simulink model "carPlant_GeHumanFollower"  (R2018b)
settings: Solver=VariableStepAuto  StartTime=0.0  StopTime=20  RelTol=1e-3
libraries: autolibshared x2, vehdynlibsteering x2
settings Model: Creator=ckreienk  LastModifiedBy=ckreienk

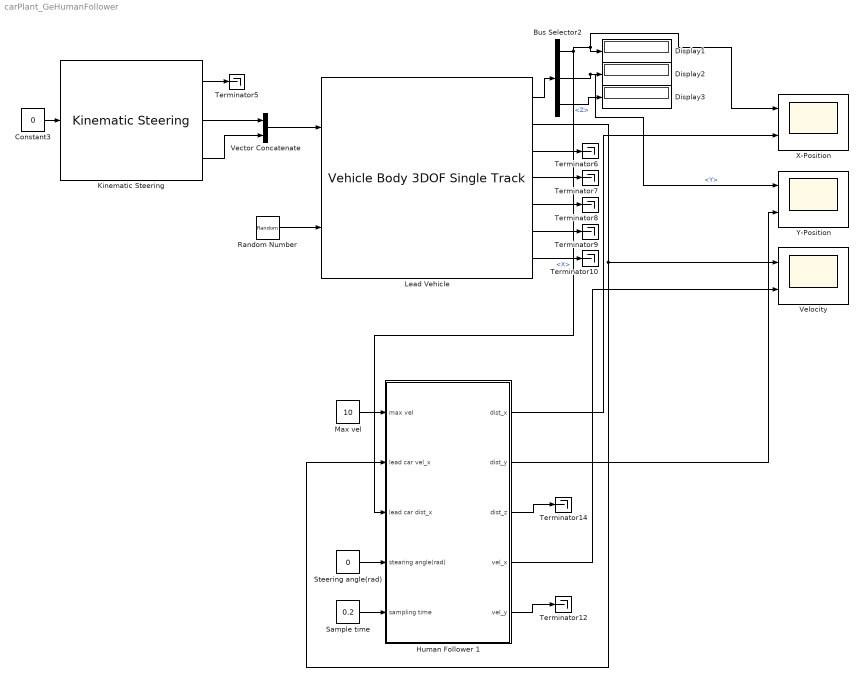
== system carPlant_GeHumanFollower ==
  Bus Selector2 : BusSelector  OutputSignals=InertFrm.Geom.Disp.X,InertFrm.Geom.Disp.Y,InertFrm.Geom.Disp.Z
  Constant3 : Constant  Value=0
  Display1 : Display
  Display2 : Display
  Display3 : Display
  Human Follower 1 : Subsystem
  Kinematic Steering : vehdynlibsteering/Kinematic Steering  StrgType=Rack and pinion  StrgRatioType=Constant  Loc=Front  NrmlFctr=0.01  TrckWdth=1  WhlBase=1.524  Db=0  StrgRng=1.25*pi  StrgAngBpts="[-6.2832   -5.0265   -3.7699   -2.5133   -1.2566         0    1.2566    2.5133    3.7699    5.0265    6.2832]"  StrgRatioTbl=|  StrgRatio=100  StrgArmLngth=0.1  RckCsLngth=0.5  TieRodLngth=0.248  D=0.2  PnnRadius=0.0057  PnnRadiusTbl="[0.0055    0.0055    0.0056    0.0057    0.0058    0.0057    0.0057    0.0057    0.0056    0.0055    0.0055]"  RodLngth=0.1  ParaArmLngth=0.9  aMode=2
      | [13.5000   13.3750   13.2500   13.1250   13.0000   13.0000   13.0000   13.1250   13.2500   13.3750   13.5000
      | ]
      settings: SourceProductName=Vehicle Dynamics Blockset
  Lead Vehicle : autolibshared/Vehicle Body 3DOF Single Track  trackMode=Dual  inputMode=External longitudinal velocity  frontSteerMode=on  rearSteerMode=off  windMode=off  muMode=off  extFMode=off  extMMode=off  aMode=2  NF=2  NR=2  m=2000  a=1.4  b=1.6  h=0.35  X_o=10  xdot_o=0  CalphaMode=off  sigmaMode=on  d=0  w=[1.4,1.4]  Cy_f=12e3  Cy_r=11e3  sigma_f=.1  sigma_r=.1  alpha_f_brk=[-.1 .1]  Cy_f_data=[-9e3 9e3]  alpha_r_brk=[-.1 .1]  Cy_r_data=[-9e3 9e3]  Y_o=0  ydot_o=0  Izz=4000  psi_o=0  r_o=0  Af=2  Cd=.3  Cl=.1  Cpm=.1  beta_w=[0:0.01:0.3]  Cs=[0:0.03:0.9]  Cym=[0:0.01:0.3]  Pabs=101325  Tair=273  g=9.81  mu=1  xdot_tol=.01  Fznom=5000  Fxtire_sat=7e4  Fytire_sat=7e4  longOff=0  latOff=0  vertOff=0
      settings: SourceProductName=Powertrain Blockset  SourceProductBaseCode=PW
  Max vel : Constant  Value=10
  Random Number : RandomNumber  Mean=3  Variance=3  SampleTime=0.1
  Sample time : Constant  Value=0.2
  Steering angle(rad) : Constant  Value=0
  Terminator{5..10,12,14} (8 alike) : Terminator
  Vector Concatenate : Concatenate
  Velocity : Scope  NumInputPorts=2
  X-Position : Scope  NumInputPorts=2
  Y-Position : Scope  NumInputPorts=2
  wires:
  Constant3/1 -> Kinematic Steering/1
  Kinematic Steering/1 -> Terminator5/1
  Kinematic Steering/2 -> Vector Concatenate/1
  Kinematic Steering/3 -> Vector Concatenate/2
  Bus Selector2/1 -> Display1/1, X-Position/1, Human Follower 1/3(lead car dist_x)  "<X>"
  Bus Selector2/2 -> Display2/1, Y-Position/1  "<Y>"
  Bus Selector2/3 -> Display3/1  "<Z>"
  Lead Vehicle/1 -> Bus Selector2/1
  Lead Vehicle/3 -> Terminator6/1
  Lead Vehicle/4 -> Terminator7/1
  Lead Vehicle/5 -> Terminator8/1
  Lead Vehicle/6 -> Terminator9/1
  Lead Vehicle/7 -> Terminator10/1
  Vector Concatenate/1 -> Lead Vehicle/1
  Random Number/1 -> Lead Vehicle/2
  Lead Vehicle/2 -> Human Follower 1/2(lead car vel_x), Velocity/1
  Sample time/1 -> Human Follower 1/5(sampling time)
  Steering angle(rad)/1 -> Human Follower 1/4(stearing angle(rad))
  Max vel/1 -> Human Follower 1/1(max vel)
  Human Follower 1/3(dist_z) -> Terminator14/1
  Human Follower 1/5(vel_y) -> Terminator12/1
  Human Follower 1/2(dist_y) -> Y-Position/2
  Human Follower 1/1(dist_x) -> X-Position/2
  Human Follower 1/4(vel_x) -> Velocity/2

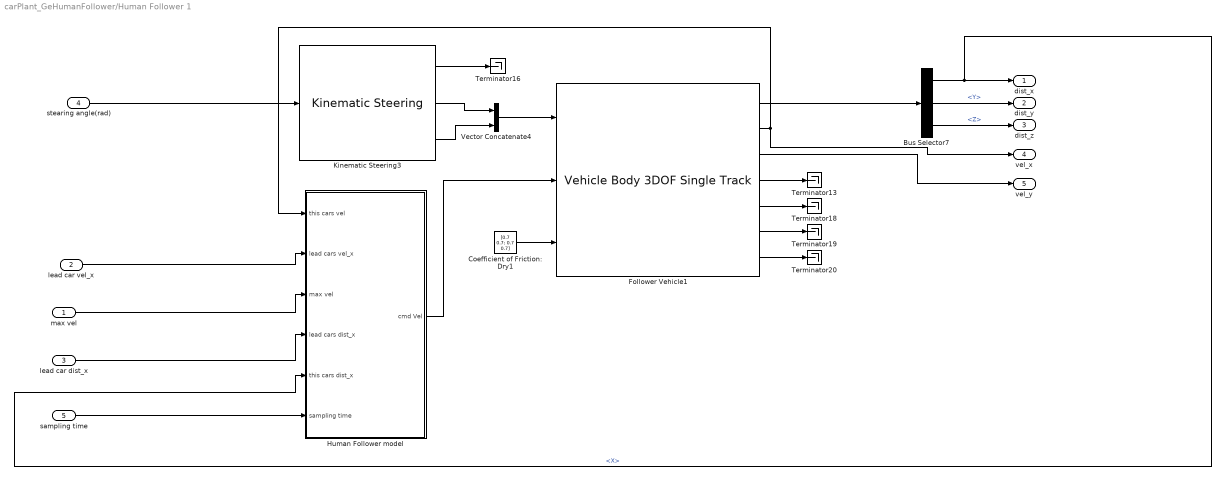
== system carPlant_GeHumanFollower/Human Follower 1 ==
  max vel : Inport
  lead car vel_x : Inport  Port=2
  lead car dist_x : Inport  Port=3
  stearing angle(rad) : Inport  Port=4
  sampling time : Inport  Port=5
  Bus Selector7 : BusSelector  OutputSignals=InertFrm.Cg.Disp.X,InertFrm.Cg.Disp.Y,InertFrm.Cg.Disp.Z
  Coefficient of Friction: Dry1 : Constant  Value=[0.7 0.7; 0.7 0.7]
  Follower Vehicle1 : autolibshared/Vehicle Body 3DOF Single Track  trackMode=Dual  inputMode=External longitudinal velocity  frontSteerMode=on  rearSteerMode=off  windMode=off  muMode=on  extFMode=off  extMMode=off  aMode=2  NF=2  NR=2  m=2000  a=1.4  b=1.6  h=0.35  X_o=0  xdot_o=0  CalphaMode=off  sigmaMode=on  d=0  w=[1.4,1.4]  Cy_f=12e3  Cy_r=11e3  sigma_f=.1  sigma_r=.1  alpha_f_brk=[-.1 .1]  Cy_f_data=[-9e3 9e3]  alpha_r_brk=[-.1 .1]  Cy_r_data=[-9e3 9e3]  Y_o=0  ydot_o=0  Izz=4000  psi_o=0  r_o=0  Af=2  Cd=.3  Cl=.1  Cpm=.1  beta_w=[0:0.01:0.3]  Cs=[0:0.03:0.9]  Cym=[0:0.01:0.3]  Pabs=101325  Tair=273  g=9.81  mu=1  xdot_tol=.01  Fznom=5000  Fxtire_sat=7e4  Fytire_sat=7e4  longOff=0  latOff=0  vertOff=0
      settings: SourceProductName=Powertrain Blockset  SourceProductBaseCode=PW
  Human Follower model : Subsystem
  Kinematic Steering3 : vehdynlibsteering/Kinematic Steering  StrgType=Rack and pinion  StrgRatioType=Constant  Loc=Front  NrmlFctr=0.01  TrckWdth=1  WhlBase=1.524  Db=0  StrgRng=1.25*pi  StrgAngBpts="[-6.2832   -5.0265   -3.7699   -2.5133   -1.2566         0    1.2566    2.5133    3.7699    5.0265    6.2832]"  StrgRatioTbl=|  StrgRatio=100  StrgArmLngth=0.1  RckCsLngth=0.5  TieRodLngth=0.248  D=0.2  PnnRadius=0.0057  PnnRadiusTbl="[0.0055    0.0055    0.0056    0.0057    0.0058    0.0057    0.0057    0.0057    0.0056    0.0055    0.0055]"  RodLngth=0.1  ParaArmLngth=0.9  aMode=2
      | [13.5000   13.3750   13.2500   13.1250   13.0000   13.0000   13.0000   13.1250   13.2500   13.3750   13.5000
      | ]
      settings: SourceProductName=Vehicle Dynamics Blockset
  Terminator{13,16,18..20} (5 alike) : Terminator
  Vector Concatenate4 : Concatenate
  dist_x : Outport
  dist_y : Outport  Port=2
  dist_z : Outport  Port=3
  vel_x : Outport  Port=4
  vel_y : Outport  Port=5
  wires:
  Bus Selector7/3 -> dist_z/1  "<Z>"
  Follower Vehicle1/5 -> Terminator18/1
  Human Follower model/1(cmd Vel) -> Follower Vehicle1/2
  max vel/1 -> Human Follower model/3(max vel)
  Follower Vehicle1/6 -> Terminator19/1
  Bus Selector7/1 -> dist_x/1, Human Follower model/5(this cars dist_x)  "<X>"
  Follower Vehicle1/4 -> Terminator13/1
  Follower Vehicle1/3 -> vel_y/1
  lead car vel_x/1 -> Human Follower model/2(lead cars vel_x)
  Follower Vehicle1/7 -> Terminator20/1
  Vector Concatenate4/1 -> Follower Vehicle1/1
  Follower Vehicle1/1 -> Bus Selector7/1
  Kinematic Steering3/1 -> Terminator16/1
  lead car dist_x/1 -> Human Follower model/4(lead cars dist_x)
  Bus Selector7/2 -> dist_y/1  "<Y>"
  sampling time/1 -> Human Follower model/6(sampling time)
  Kinematic Steering3/2 -> Vector Concatenate4/1
  stearing angle(rad)/1 -> Kinematic Steering3/1
  Kinematic Steering3/3 -> Vector Concatenate4/2
  Follower Vehicle1/2 -> Human Follower model/1(this cars vel), vel_x/1
  Coefficient of Friction: Dry1/1 -> Follower Vehicle1/3

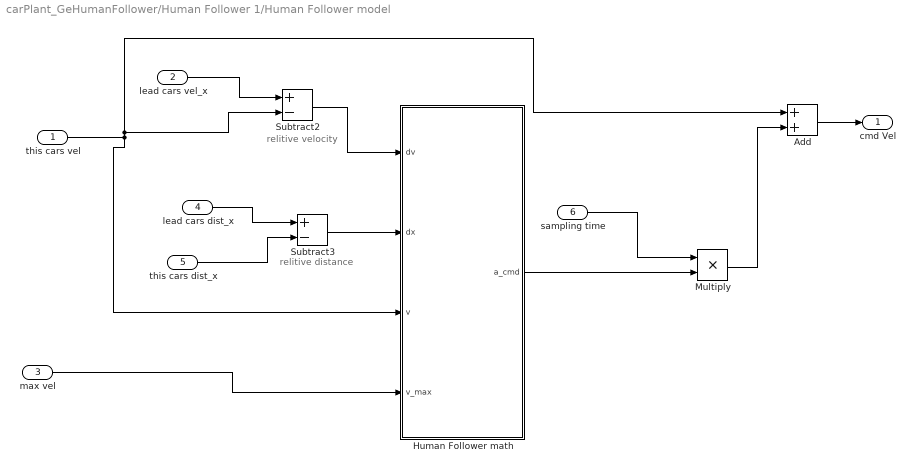
== system carPlant_GeHumanFollower/Human Follower 1/Human Follower model ==
  note: relitive distance
  note: relitive velocity
  this cars vel : Inport
  lead cars vel_x : Inport  Port=2
  max vel : Inport  Port=3
  lead cars dist_x : Inport  Port=4
  this cars dist_x : Inport  Port=5
  sampling time : Inport  Port=6
  Add : Sum
  Human Follower math : Subsystem
  Multiply : Product
  Subtract2 : Sum  Inputs=+-
  Subtract3 : Sum  Inputs=+-
  cmd Vel : Outport
  wires:
  Add/1 -> cmd Vel/1
  lead cars dist_x/1 -> Subtract3/1
  this cars vel/1 -> Human Follower math/3(v), Add/1, Subtract2/2
  Human Follower math/1(a_cmd) -> Multiply/2
  Subtract3/1 -> Human Follower math/2(dx)
  Multiply/1 -> Add/2
  this cars dist_x/1 -> Subtract3/2
  Subtract2/1 -> Human Follower math/1(dv)
  max vel/1 -> Human Follower math/4(v_max)
  sampling time/1 -> Multiply/1
  lead cars vel_x/1 -> Subtract2/1

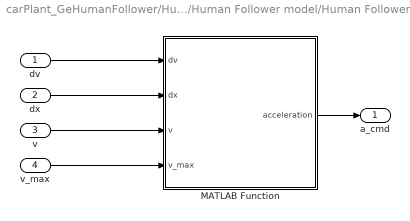
== system carPlant_GeHumanFollower/Human Follower 1/Human Follower model/Human Follower math ==
  dv : Inport
  dx : Inport  Port=2
  v : Inport  Port=3
  v_max : Inport  Port=4
  MATLAB Function : MATLAB Function  TreatAsAtomicUnit=on
  a_cmd : Outport
  wires:
  v_max/1 -> MATLAB Function/4(v_max)
  MATLAB Function/1(acceleration) -> a_cmd/1
  v/1 -> MATLAB Function/3(v)
  dv/1 -> MATLAB Function/1(dv)
  dx/1 -> MATLAB Function/2(dx)

== matlab function carPlant_GeHumanFollower/Human Follower 1/Human Follower model/Human Follower math/MATLAB Function ==
  data: dv input; dx input; v input; v_max input; acceleration output
function acceleration = fcn(dv, dx, v, v_max)

if dx <= 10
    V = 0;
elseif dx <= 35
    V = dx - 10;
else
    V = 30;
end

if dv + v <= v_max
    w = v + dv;
else
    w = v_max;
end

acceleration = 0.1*(V-v) + 0.5*(w-v);
